simulink model "test4_1"  (R2024b)
settings: Solver=VariableStepAuto  StartTime=0.0  StopTime=10.0  RelTol=1e-3
values from neighbouring files (symbols this model uses):
  A = [(-cy.f-cy.r)/(m*Vx),(-l.f*cy.f+l.r*cy.r)/(m*Vx)-Vx;(-l.f*cy.f+l.r*cy.r)/(Izz*Vx),(-l.f^2*cy.f-l.r^2*cy.r)/(Izz*Vx)]    [test4_1.m]    (also in untitled1.m = [(-cy.f-cy.r)/(m*Vx),(-lf*cy.f+lr*cy.r)/(m*Vx)-Vx;(-lf*cy.f+)
  B = [cy.f/(m*Vx);(l.f*cy.f)/Izz]    [test4_1.m]    (also in untitled1.m = [cy.f/(m*Vx);(lf*cy.f)/Izz])
  C = [1,0;0,1]    [test4_1.m]    (also in untitled1.m)
  D = [0;0]    [test4_1.m]    (also in untitled1.m)
settings Model: Creator=lijiy  LastModifiedBy=lijiy

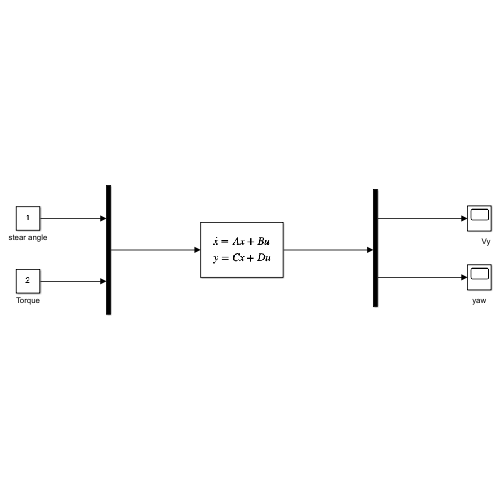
[thumbnail: Simulink's stored preview of the top-level diagram]
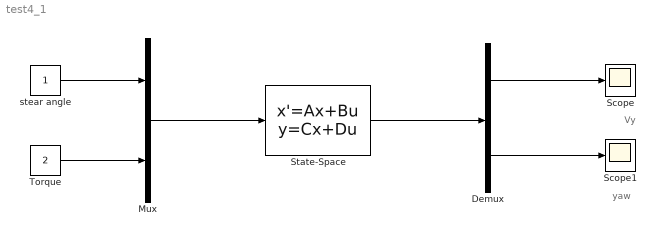
== system test4_1 ==
  note: yaw
  note: Vy
  Demux : Demux  Outputs=2
  Mux : Mux  Inputs=2
  Scope : Scope
  Scope1 : Scope
  State-Space : StateSpace  A=A  B=B  C=C  D=D  InitialCondition=0
  Torque : Constant  Value=2
  stear angle : Constant
  wires:
  Mux/1 -> State-Space/1
  stear angle/1 -> Mux/1
  Torque/1 -> Mux/2
  State-Space/1 -> Demux/1
  Demux/2 -> Scope1/1
  Demux/1 -> Scope/1
